simulink model "Lab6_1"  (R2016a)
settings: Solver=FixedStepDiscrete  StartTime=0.0  StopTime=10.0  RelTol=1e-3
settings Model: Creator=NoteBook  LastModifiedBy=NoteBook
settings OptimizationCC: DefaultParameterBehavior=Inlined  EnableMemcpy=off  OptimizeModelRefInitCode=on  LifeSpan=1
settings DebuggingCC: UnderspecifiedInitializationDetection=Classic  MergeDetectMultiDrivingBlocksExec=none
settings ModelReferenceCC: PropagateSignalLabelsOutOfModel=off
settings RTWCC: SystemTargetFile=ert.tlc  GenCodeOnly=on  TemplateMakefile=ert_default_tmf  GenerateReport=on  IncludeHyperlinkInReport=on  LaunchReport=on  GenerateTraceInfo=on  GenerateTraceReport=on  GenerateTraceReportSl=on  GenerateTraceReportSf=on  GenerateTraceReportEml=on
settings CodeAppCC: ForceParamTrailComments=on  IgnoreCustomStorageClasses=off  OperatorAnnotations=on  SimulinkDataObjDesc=on  SFDataObjDesc=on  MATLABFcnDesc=on  InsertBlockDesc=on  MATLABSourceComments=on
settings ERTTargetCC: GenerateSampleERTMain=on  InlinedParameterPlacement=NonHierarchical  ERTCustomFileTemplate=example_file_process.tlc

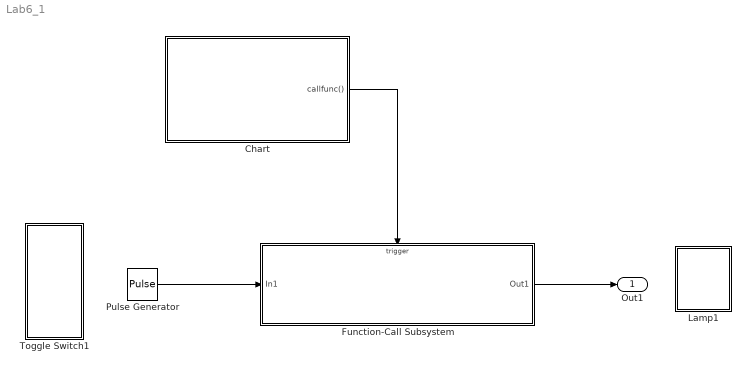
== system Lab6_1 ==
  Chart : Stateflow chart  TreatAsAtomicUnit=on
  Function-Call Subsystem : Subsystem  TreatAsAtomicUnit=on
  Lamp1 : Subsystem  DialogController=hmiCreateDDGDialog  IsWebBlock=on  mask(MWDashboardBlock){webBlockId=e22f5acb-ac90-437b-b799-f96cc2329583, webBlockType=lamp, ShowInLibBrowser=on, ShowInitialText=on, HMISrcModelName=Lab6_1}
      mask prompts: webBlockType "WebBlock Type"; HMISrcModelName "Source Model"
      mask Help: helpview([docroot '/mapfiles/simulink.map'], 'hmi_lamp')
      mask Display:
      | if strcmp(get_param(bdroot(gcb),'BlockDiagramType'), 'library')
      |     image([(matlabroot) '/toolbox/simulink/hmi/icons/Lamp.png']);
      | end
  Pulse Generator : DiscretePulseGenerator  PulseType=Time based  Amplitude=0  Period=10  PulseWidth=5
  Toggle Switch1 : Subsystem  DialogController=hmiCreateDDGDialog  IsWebBlock=on  mask(MWDashboardBlock){webBlockId=aeb6cdb8-defc-4816-a0d5-acb31be90235, webBlockType=toggleswitch, ShowInLibBrowser=on, ShowInitialText=on, HMISrcModelName=Lab6_1}
      mask prompts: webBlockId "WebBlock Id"; webBlockType "WebBlock Type"; HMISrcModelName "Source Model"
      mask Help: helpview([docroot '/mapfiles/simulink.map'], 'hmi_toggle_switch')
      mask Display:
      | if strcmp(get_param(bdroot(gcb),'BlockDiagramType'), 'library')
      |     image([(matlabroot) '/toolbox/simulink/hmi/icons/ToggleSwitch.png']);
      | end
  Out1 : Outport
  wires:
  Function-Call Subsystem/1(Out1) -> Out1/1
  Chart/1(callfunc()) -> Function-Call Subsystem/Trigger
  Pulse Generator/1 -> Function-Call Subsystem/1(In1)

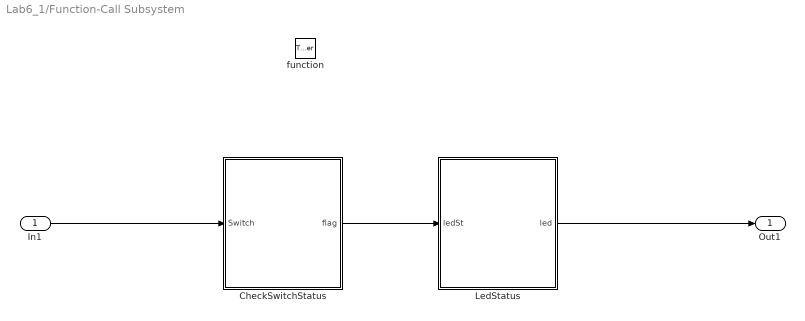
== system Lab6_1/Function-Call Subsystem ==
  In1 : Inport
  function : TriggerPort  TriggerType=function-call  VariantControl=Variant
  CheckSwitchStatus : Stateflow chart  TreatAsAtomicUnit=on
  "LedStatus " : Stateflow chart  TreatAsAtomicUnit=on
  Out1 : Outport
  wires:
  In1/1 -> CheckSwitchStatus/1(Switch)
  CheckSwitchStatus/1(flag) -> "LedStatus "/1(ledSt)
  "LedStatus "/1(led) -> Out1/1

== system Lab6_1/Lamp1 ==

== system Lab6_1/Toggle Switch1 ==

== stateflow chart Lab6_1/Function-Call Subsystem/LedStatus  ==
  (default) -> (junction 7) : % LedStatus
  (junction 7) -> (junction 8) [order 1] : [ledSt == 1]
  (junction 7) -> (junction 9) [order 2] : {led = 0;}
  (junction 8) -> (junction 10) : {led = 1;}
  (junction 10) -> (junction 9)
  (junction 9) -> (junction 11)
  data: ledSt input; led output

== stateflow chart Lab6_1/Chart ==
  state Call_Fuction
    en:
    du:
    ex:
  (default) -> Call_Fuction
  Call_Fuction -> Call_Fuction : [after(5,msec)]{callfunc;}
  events: callfunc output FUNCTION_CALL_EVENT

== stateflow chart Lab6_1/Function-Call Subsystem/CheckSwitchStatus ==
  (default) -> (junction 7) : % Check Button
  (junction 7) -> (junction 8) [order 1] : [Switch == 1]
  (junction 7) -> (junction 9) [order 2] : {flag = 0;}
  (junction 8) -> (junction 10) : {flag = 1;}
  (junction 10) -> (junction 9)
  (junction 9) -> (junction 11)
  data: Switch input; flag output
